simulink model "PRIM_TFnumbers_BZY2DH"  (R2017a)
settings: Solver=VariableStepAuto  StartTime=0.0  StopTime=10.0  RelTol=1e-3
undefined symbols (not defined in the file): Ed, Ts, Ts_Control, Ts_Pw, Ts_sf
libraries: simulink x2, powerlib_extras x1
settings Model: Creator=BZy  LastModifiedBy=BZy

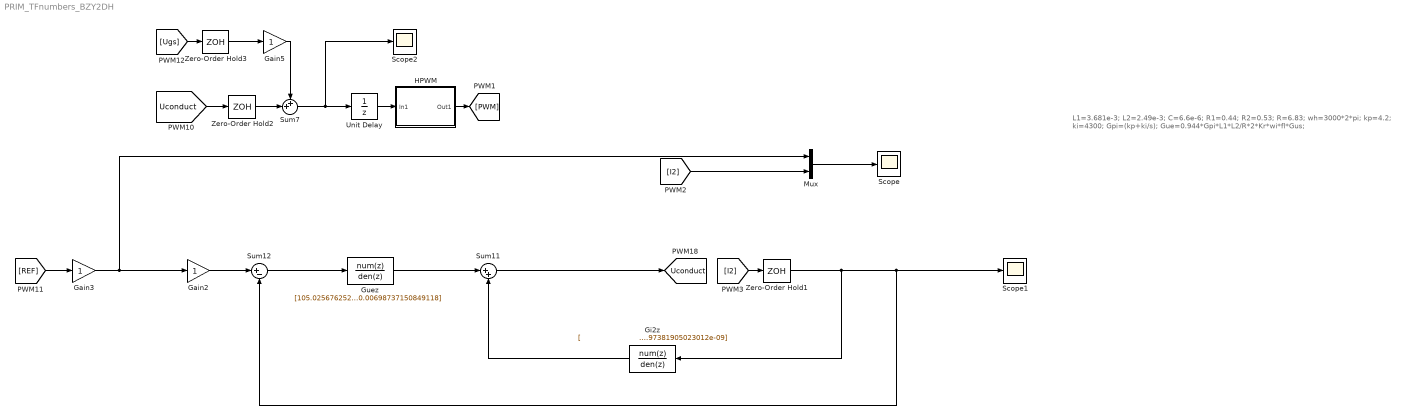
== system PRIM_TFnumbers_BZY2DH ==
  note: L1=3.681e-3;
      | L2=2.49e-3;
      | C=6.6e-6;
      | R1=0.44;
      | R2=0.53;
      | R=6.83;
      | wh=3000*2*pi;
      |
      | kp=4.2;
      | ki=4300;
      | Gpi=(kp+ki/s);
      | Gue=0.944*Gpi*L1*L2/R*2*Kr*wi*fl*Gus;
  Gain2 : Gain
  Gain3 : Gain
  Gain5 : Gain
  Gi2z : DiscreteTransferFcn  Numerator="[                         0          19.2644080939765          -151.38298327259          550.190243428913         -1225.88011101113          1868.13692864995         -2051.09208109317          1655.79378318097         -972.521670074443          386.057598385935          -69.062063595164         -30.5863874120469          32.9237004112229         -16.1038727451287          5.36844286878031         -1.31852049632393         0.242695623706439       -0.0331645722320292       0.00326081599524444     -0.000216958116484304      8.65468730110477e-06     -1.53211927855947e-07]"  Denominator="[                        1         -8.26254583308024          32.3259000555758         -79.7202886298294          139.142089195404         -182.893822093046          188.048197920109         -155.034648672193          104.207346345468         -57.7396920380286          26.5542416124631         -10.1708145436179          3.24535772084055        -0.860241324079864          0.18823332859043       -0.0336463999128626       0.00483471296496897     -0.000545105874986923      4.64564316052198e-05     -2.81420889523269e-06      1.07998488512359e-07     -1.97381905023012e-09]"  SampleTime=Ts
  Guez : DiscreteTransferFcn  Numerator="[105.025676252564         -276.476408871867          271.352053418996         -124.664250921948          27.6326778785761         -2.42740799538648]"  Denominator="[                         1          -2.0279676350747          1.46208101400042        -0.522532820057753        0.0954068126405283      -0.00698737150849118]"  SampleTime=Ts
  HPWM : Subsystem
  Mux : Mux  Inputs=2
  Scope : Scope
  Scope1 : Scope
  Scope2 : Scope
  Sum11 : Sum  Inputs=|++
  Sum12 : Sum  Inputs=|+-
  Sum7 : Sum  Inputs=++|
  Unit Delay : UnitDelay  InitialCondition=1  SampleTime=Ts_Control
  Zero-Order Hold1 : ZeroOrderHold  SampleTime=Ts_Control
  Zero-Order Hold2 : ZeroOrderHold  SampleTime=Ts_Control
  Zero-Order Hold3 : ZeroOrderHold  SampleTime=Ts_Control
  tag scope: Uconduct=global
  wires:
  [Uconduct] -> Zero-Order Hold2/1
  Gain5/1 -> Sum7/1
  Sum7/1 -> Unit Delay/1, Scope2/1
  [Ugs] -> Zero-Order Hold3/1
  HPWM/1(Out1) -> [PWM]
  Zero-Order Hold2/1 -> Sum7/2
  Unit Delay/1 -> HPWM/1(In1)
  Zero-Order Hold3/1 -> Gain5/1
  Gain3/1 -> Mux/1, Gain2/1
  Gain2/1 -> Sum12/1
  Mux/1 -> Scope/1
  [I2] -> Zero-Order Hold1/1
  [REF] -> Gain3/1
  Zero-Order Hold1/1 -> Gi2z/1, Sum12/2, Scope1/1
  [I2] -> Mux/2
  Gi2z/1 -> Sum11/2
  Sum11/1 -> [Uconduct]
  Guez/1 -> Sum11/1
  Sum12/1 -> Guez/1

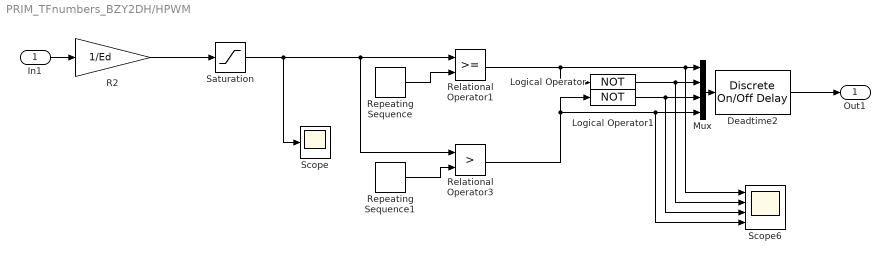
== system PRIM_TFnumbers_BZY2DH/HPWM ==
  In1 : Inport
  Deadtime2 : powerlib_extras/Discrete  Control Blocks/Discrete On//Off Delay  type_delay=On delay  delay=3.2e-6  ic=0  Ts=Ts_Pw
  Logical Operator : Logic  Operator=NOT  AllPortsSameDT=off  OutDataTypeStr=boolean
  Logical Operator1 : Logic  Operator=NOT  AllPortsSameDT=off  OutDataTypeStr=boolean
  Mux : Mux
  R2 : Gain  Gain=1/Ed  SaturateOnIntegerOverflow=on  OutDataTypeStr=Inherit: Same as input  ParamDataTypeStr=Inherit: Same as input
  Relational Operator1 : RelationalOperator  OutDataTypeStr=boolean  SampleTime=Ts_Pw  RndMeth=Nearest
  Relational Operator3 : RelationalOperator  Operator=>  OutDataTypeStr=boolean  SampleTime=Ts_Pw  RndMeth=Nearest
  Repeating Sequence : simulink/Sources/Repeating Sequence  rep_seq_t="[0 Ts_sf/2  Ts_sf]"  rep_seq_y=[0 1 0]
  Repeating Sequence1 : simulink/Sources/Repeating Sequence  rep_seq_t="[0 Ts_sf/2  Ts_sf]"  rep_seq_y=[0 -1 0]
  Saturation : Saturate  UpperLimit=0.95  LowerLimit=-0.95
  Scope : Scope
  Scope6 : Scope  NumInputPorts=4
  Out1 : Outport
  wires:
  Logical Operator/1 -> Mux/2, Scope6/2
  Mux/1 -> Deadtime2/1
  In1/1 -> R2/1
  Repeating Sequence/1 -> Relational Operator1/2
  Relational Operator1/1 -> Logical Operator/1, Mux/1, Scope6/1
  Repeating Sequence1/1 -> Relational Operator3/2
  Relational Operator3/1 -> Logical Operator1/1, Mux/4, Scope6/4
  Logical Operator1/1 -> Mux/3, Scope6/3
  R2/1 -> Saturation/1
  Deadtime2/1 -> Out1/1
  Saturation/1 -> Scope/1, Relational Operator3/1, Relational Operator1/1
